simulink library "lib_transmission2"  (Simulink 10.1)
settings: Solver=VariableStepAuto  StartTime=0.0  StopTime=10.0  RelTol=1e-3
undefined symbols (not defined in the file or in its folder): cyc_mph, fc_map_spd, fc_max_trq, fc_spd_scale, fc_trq_scale, fd_inertia, fd_loss, fd_ratio, gb_gear_number_lookup, gb_gears_num, gb_inertia, gb_loss_const, gb_loss_input_spd_coeff, gb_loss_input_trq_coeff, gb_loss_output_spd_coeff, gb_loss_output_trq_coeff, gb_num_init, gb_ratio, gb_shift_delay, gb_spd_scale, gb_trq_scale, htc_inertia, htc_k_adv, htc_k_adv_coast, htc_lockup, htc_lockup_load, htc_lockup_spd, htc_lu_gear_range, htc_max_coast_tr, htc_min_coast_tr, htc_pump_loss_spd, htc_pump_loss_trq_lockup, htc_pump_loss_trq_unlock, htc_sr, htc_sr_coast, htc_tr, htc_tr_coast, htc_unlock_spd, mc_map_spd, mc_max_trq, mc_overtrq_factor, mc_spd_scale, mc_trq_scale, tc_loss, tc_mc_to_fc_ratio, tx_eff_map, tx_map_spd, tx_map_trq, tx_pg_r, tx_pg_s, tx_speed_dep, vc_clutch_bool, vc_idle_spd, vc_launch_spd, wh_radius
undefined symbols (not defined in the file): gb_dnshift_load, gb_dnshift_spd, gb_map_spd_out, gb_map_trq_in, gb_map_trq_out, gb_upshift_load, gb_upshift_spd, logFlag
libraries: lib_controls x1, lib_etc x1, lib_controls2 x1, lib_transmission x1
(part 14 of 17)

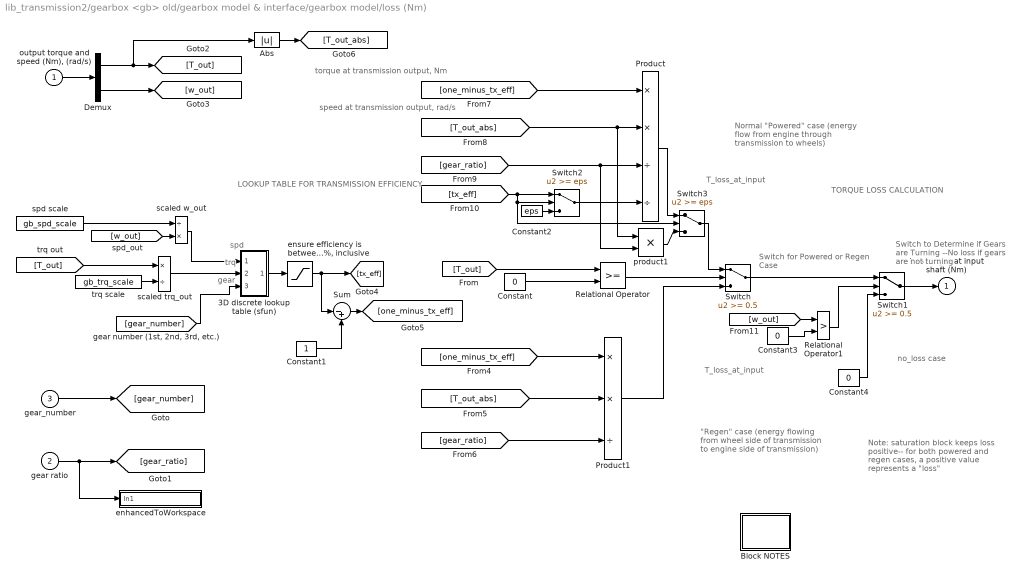
== system lib_transmission2/gearbox <gb> old/gearbox model & interface/gearbox model/loss (Nm) ==
  note: TORQUE LOSS CALCULATION
  note: gear
  note: trq
  note: spd
  note: torque at transmission output, Nm
  note: speed at transmission output, rad/s
  note: no_loss case
  note: Note: saturation block keeps
      | loss positive-- for both powered
      | and regen cases, a
      | positive value represents a "loss"
  note: Switch for Powered
      |  or Regen Case
  note: Switch to Determine
      | if Gears are Turning
      | --No loss if gears
      | are not turning
  note: Normal "Powered" case
      | (energy flow from engine
      | through transmission to wheels)
  note: T_loss_at_input
  note: "Regen" case
      | (energy flowing from
      | wheel side of transmission
      | to engine side of transmission)
  note: T_loss_at_input
  note: LOOKUP TABLE FOR TRANSMISSION EFFICIENCY
  "output torque and speed (Nm), (rad/s)" : Inport
  gear ratio : Inport  Port=2
  gear_number : Inport  Port=3
  3D discrete lookup table (sfun) : Subsystem  mask{tx_map_spd=tx_map_spd, tx_map_trq=tx_map_trq, tx_eff_map=tx_eff_map}
      mask prompts: tx_map_spd "Row Lookup"; tx_map_trq "Column Lookup"; tx_eff_map "Lookup Matrix"
  Abs : Abs  SaturateOnIntegerOverflow=on
  Block NOTES : Subsystem
      mask Display: disp('Block\nNOTES')
  Constant : Constant  Value=0
  Constant1 : Constant
  Constant2 : Constant  Value=eps
  Constant3 : Constant  Value=0
  Constant4 : Constant  Value=0
  Demux : Demux  Outputs=2
  Product : Product  Inputs=**//  SaturateOnIntegerOverflow=on
  Product1 : Product  Inputs=**/  SaturateOnIntegerOverflow=on
  Relational Operator : RelationalOperator  RndMeth=Nearest  InputSameDT=on
  Relational Operator1 : RelationalOperator  Operator=>  RndMeth=Nearest  InputSameDT=on
  Sum : Sum  Inputs=|-+  SaturateOnIntegerOverflow=on
  Switch : Switch  Threshold=0.5  SaturateOnIntegerOverflow=on  InputSameDT=on
  Switch1 : Switch  Threshold=0.5  SaturateOnIntegerOverflow=on  InputSameDT=on
  Switch2 : Switch  Threshold=eps  SaturateOnIntegerOverflow=on  InputSameDT=on
  Switch3 : Switch  Threshold=eps  SaturateOnIntegerOverflow=on  InputSameDT=on
  enhancedToWorkspace : Subsystem  TreatAsAtomicUnit=on  mask(enhancedToWorkspace){generalName=generalName, specificName=current_gear_ratio, logFlag=logFlag}
      mask prompts: generalName "General Name [char-evaluated]"; specificName "Specific Name [char-literal]"; logFlag "Enable flag (1=on,0=off)"
      mask help: A wrapper for the Simulink "To Workspace" block that allows you to evaluate the name of the variable to log to workspace. This is useful to avoid the double logging errors that occur when you pull in two library models that attempt to log to the same variable.
      mask init:
      | enhancedToWsMaker
      settings: CopyFcn=breakLinkCopyFcn  ParentCloseFcn=breakLinkParCloseFcn
      mask Help:
      | <h2>Enhanced To Workspace Block</h2>
      | <h3>Parameters</h3>
      | <UL>
      | <li><b>General Name:</b> This is the more general name of the variable. Variables are saved to the workspace as <i>generalName_specificName</i>. Note that this is an evaluated variable. If you would like to type in the value directly, it must be surrounded with single quotes. Otherwise you can input the name of a variable containing a char string.</li>
      | <li><b>Specific Name:</b> This is the specific name of the variable. Note that this is input as a char literal (i.e., you don't need quotes).</li>
      | <li><b>Enable Flag:</b> This flag should have the value of 0 or 1. If 0, the variable will not be logged to the workspace. If 1, the variable will be logged. This is done so that variable logging can be turned off to improve speed.</li>
      | </ul>
      | <h3>Overview</h3>
      | <p>The enhanced to workspace block was put together to allow one to dynamically resolve variable names at run time in simulink. This is most powerful when used in conjunction with a masked subsystem to allow multiple instances of that masked subsytem to be used in the same model. The strategy is to set the generalName in the block mask which will allow the block to change the general name for all variable logging on the fly.
      | <h3>Helper Files</h3>
      | <p>Three m-files are required by the enhancedToWorkspace block. These files are located in the &lt; ADVISOR root &gt;/GUI directory :
      | <ul>
      | <li><i>enhancedToWsMaker.m</i> This file runs the mask initialization for the block</li>
      | <li><i>breakLinkCopyFcn.m</i> This file is used by the block callback when the simulink block is copied. It is necessary to break the link to the enhancedToWorkspace similar to the To Workspace block in order for it to be able to configure itself. (Try copying simulink's To Workspace block--it is impossible to make a link)</li>
      | <li><i>breakLinkParCloseFcn.m</i> This file is similar to the breakLinkCopyFcn and is used when a parent system is closed</li>
      | </ul>
      | <hr>
      | 
      | <p>Created 2003-Jan-21, Michael Patrick O'Keefe, NREL</p>
      | 
      | <!--
      | <VARDEF>
      | <H3>var_name</H3>
      | <UL>
      | <LI><B>data type</B> data type here</LI>
      | <LI><B>units</B> units here</LI>
      | <LI><B>vehicle type</B> vehicle type here</LI>
      | <LI><B>description</B> description here</LI>
      | </UL>
      | </VARDEF>
      | -->
      mask Display: disp([generalName,'_',specificName])
  "ensure efficiency is between  0% and 100%, inclusive" : Saturate  UpperLimit=1  LowerLimit=0
  product1 : Product  SaturateOnIntegerOverflow=on
  scaled trq_out : Product  Inputs=*/  SaturateOnIntegerOverflow=on
  scaled w_out : Product  Inputs=/*  SaturateOnIntegerOverflow=on
  spd scale : Constant  Value=gb_spd_scale
  trq scale : Constant  Value=gb_trq_scale
  loss torque at input shaft (Nm) : Outport  InitialOutput=0
  wires:
  product1/1 -> Switch3/3
  Product/1 -> Switch3/1
  Switch3/1 -> Switch/1
  Constant2/1 -> Switch2/3
  [tx_eff] -> Switch3/2, Switch2/2, Switch2/1
  Switch2/1 -> Product/4
  gear_number/1 -> [gear_number]
  gear ratio/1 -> [gear_ratio], enhancedToWorkspace/1(In1)
  spd scale/1 -> scaled w_out/1
  [w_out] -> scaled w_out/2
  Sum/1 -> [one_minus_tx_eff]
  Constant1/1 -> Sum/2
  trq scale/1 -> scaled trq_out/2
  scaled trq_out/1 -> 3D discrete lookup table (sfun)/2(lookup trq (Nm))
  [T_out] -> scaled trq_out/1
  scaled w_out/1 -> 3D discrete lookup table (sfun)/1(lookup speed (rad/s))
  "ensure efficiency is between  0% and 100%, inclusive"/1 -> Sum/1, [tx_eff]
  3D discrete lookup table (sfun)/1(tx_eff) -> "ensure efficiency is between  0% and 100%, inclusive"/1
  Switch/1 -> Switch1/1
  Abs/1 -> [T_out_abs]
  Demux/1 -> Abs/1, [T_out]
  Relational Operator1/1 -> Switch1/2
  Constant3/1 -> Relational Operator1/2
  [w_out] -> Relational Operator1/1
  Constant4/1 -> Switch1/3
  Switch1/1 -> loss torque at input shaft (Nm)/1
  [gear_ratio] -> product1/2, Product/3
  [T_out_abs] -> product1/1, Product/2
  [one_minus_tx_eff] -> Product/1
  [T_out_abs] -> Product1/2
  [gear_ratio] -> Product1/3
  [one_minus_tx_eff] -> Product1/1
  Product1/1 -> Switch/3
  [T_out] -> Relational Operator/1
  Constant/1 -> Relational Operator/2
  Relational Operator/1 -> Switch/2
  [gear_number] -> 3D discrete lookup table (sfun)/3("gear_number  (e.g., 1, 2, 3)")
  Demux/2 -> [w_out]
  "output torque and speed (Nm), (rad/s)"/1 -> Demux/1

== system lib_transmission2/hydraulic torque converter <htc>/conventional HTC  and Interface/htc model/SR ==
  T,w req out : Inport
  w in : Inport  Port=2
  >0 : Saturate  UpperLimit=inf  LowerLimit=eps
  Constant : Constant  Value=0
  Constant1 : Constant  Value=vc_idle_spd+eps
  Constant3 : Constant
  K_adv : Subsystem
  K_adv_coast : Subsystem
  Logical Operator : Logic  Operator=NOT  Inputs=1
  Logical Operator1 : Logic  Operator=NOT  Inputs=1
  MinMax : MinMax  Inputs=2
  Relational Operator : RelationalOperator  RndMeth=Nearest  InputSameDT=on
  SR Look-Up Table SR=wout/win : Lookup  InputValues=htc_k_adv  Table=htc_sr  SaturateOnIntegerOverflow=on
  SR Look-Up Table SR=wout/win coast : Lookup  InputValues=fliplr(htc_k_adv_coast)  Table=fliplr(htc_sr_coast)  SaturateOnIntegerOverflow=on
  SRmax= wout/win,min : Product  Inputs=*/  SaturateOnIntegerOverflow=on
  T : Selector  InputPortWidth=2  IndexOptions=Index vector (dialog)  Indices=1  OutputSizes=1
  enhancedToWorkspace1 : Subsystem  TreatAsAtomicUnit=on  mask(enhancedToWorkspace){generalName=generalName, specificName=coasting, logFlag=logFlag}
      mask prompts: generalName "General Name [char-evaluated]"; specificName "Specific Name [char-literal]"; logFlag "Enable flag (1=on,0=off)"
      mask help: A wrapper for the Simulink "To Workspace" block that allows you to evaluate the name of the variable to log to workspace. This is useful to avoid the double logging errors that occur when you pull in two library models that attempt to log to the same variable.
      mask init:
      | enhancedToWsMaker
      settings: CopyFcn=breakLinkCopyFcn  ParentCloseFcn=breakLinkParCloseFcn
      mask Help:
      | <h2>Enhanced To Workspace Block</h2>
      | <h3>Parameters</h3>
      | <UL>
      | <li><b>General Name:</b> This is the more general name of the variable. Variables are saved to the workspace as <i>generalName_specificName</i>. Note that this is an evaluated variable. If you would like to type in the value directly, it must be surrounded with single quotes. Otherwise you can input the name of a variable containing a char string.</li>
      | <li><b>Specific Name:</b> This is the specific name of the variable. Note that this is input as a char literal (i.e., you don't need quotes).</li>
      | <li><b>Enable Flag:</b> This flag should have the value of 0 or 1. If 0, the variable will not be logged to the workspace. If 1, the variable will be logged. This is done so that variable logging can be turned off to improve speed.</li>
      | </ul>
      | <h3>Overview</h3>
      | <p>The enhanced to workspace block was put together to allow one to dynamically resolve variable names at run time in simulink. This is most powerful when used in conjunction with a masked subsystem to allow multiple instances of that masked subsytem to be used in the same model. The strategy is to set the generalName in the block mask which will allow the block to change the general name for all variable logging on the fly.
      | <h3>Helper Files</h3>
      | <p>Three m-files are required by the enhancedToWorkspace block. These files are located in the &lt; ADVISOR root &gt;/GUI directory :
      | <ul>
      | <li><i>enhancedToWsMaker.m</i> This file runs the mask initialization for the block</li>
      | <li><i>breakLinkCopyFcn.m</i> This file is used by the block callback when the simulink block is copied. It is necessary to break the link to the enhancedToWorkspace similar to the To Workspace block in order for it to be able to configure itself. (Try copying simulink's To Workspace block--it is impossible to make a link)</li>
      | <li><i>breakLinkParCloseFcn.m</i> This file is similar to the breakLinkCopyFcn and is used when a parent system is closed</li>
      | </ul>
      | <hr>
      | 
      | <p>Created 2003-Jan-21, Michael Patrick O'Keefe, NREL</p>
      | 
      | <!--
      | <VARDEF>
      | <H3>var_name</H3>
      | <UL>
      | <LI><B>data type</B> data type here</LI>
      | <LI><B>units</B> units here</LI>
      | <LI><B>vehicle type</B> vehicle type here</LI>
      | <LI><B>description</B> description here</LI>
      | </UL>
      | </VARDEF>
      | -->
      mask Display: disp([generalName,'_',specificName])
  enhancedToWorkspace2 : Subsystem  TreatAsAtomicUnit=on  mask(enhancedToWorkspace){generalName=generalName, specificName=locked, logFlag=logFlag}
      mask prompts: generalName "General Name [char-evaluated]"; specificName "Specific Name [char-literal]"; logFlag "Enable flag (1=on,0=off)"
      mask help: A wrapper for the Simulink "To Workspace" block that allows you to evaluate the name of the variable to log to workspace. This is useful to avoid the double logging errors that occur when you pull in two library models that attempt to log to the same variable.
      mask init:
      | enhancedToWsMaker
      settings: CopyFcn=breakLinkCopyFcn  ParentCloseFcn=breakLinkParCloseFcn
      mask Help:
      | <h2>Enhanced To Workspace Block</h2>
      | <h3>Parameters</h3>
      | <UL>
      | <li><b>General Name:</b> This is the more general name of the variable. Variables are saved to the workspace as <i>generalName_specificName</i>. Note that this is an evaluated variable. If you would like to type in the value directly, it must be surrounded with single quotes. Otherwise you can input the name of a variable containing a char string.</li>
      | <li><b>Specific Name:</b> This is the specific name of the variable. Note that this is input as a char literal (i.e., you don't need quotes).</li>
      | <li><b>Enable Flag:</b> This flag should have the value of 0 or 1. If 0, the variable will not be logged to the workspace. If 1, the variable will be logged. This is done so that variable logging can be turned off to improve speed.</li>
      | </ul>
      | <h3>Overview</h3>
      | <p>The enhanced to workspace block was put together to allow one to dynamically resolve variable names at run time in simulink. This is most powerful when used in conjunction with a masked subsystem to allow multiple instances of that masked subsytem to be used in the same model. The strategy is to set the generalName in the block mask which will allow the block to change the general name for all variable logging on the fly.
      | <h3>Helper Files</h3>
      | <p>Three m-files are required by the enhancedToWorkspace block. These files are located in the &lt; ADVISOR root &gt;/GUI directory :
      | <ul>
      | <li><i>enhancedToWsMaker.m</i> This file runs the mask initialization for the block</li>
      | <li><i>breakLinkCopyFcn.m</i> This file is used by the block callback when the simulink block is copied. It is necessary to break the link to the enhancedToWorkspace similar to the To Workspace block in order for it to be able to configure itself. (Try copying simulink's To Workspace block--it is impossible to make a link)</li>
      | <li><i>breakLinkParCloseFcn.m</i> This file is similar to the breakLinkCopyFcn and is used when a parent system is closed</li>
      | </ul>
      | <hr>
      | 
      | <p>Created 2003-Jan-21, Michael Patrick O'Keefe, NREL</p>
      | 
      | <!--
      | <VARDEF>
      | <H3>var_name</H3>
      | <UL>
      | <LI><B>data type</B> data type here</LI>
      | <LI><B>units</B> units here</LI>
      | <LI><B>vehicle type</B> vehicle type here</LI>
      | <LI><B>description</B> description here</LI>
      | </UL>
      | </VARDEF>
      | -->
      mask Display: disp([generalName,'_',specificName])
  if coasting : Switch  Threshold=eps  SaturateOnIntegerOverflow=on  InputSameDT=on
  "locked up, then SR=1" : Switch  Threshold=eps  SaturateOnIntegerOverflow=on  InputSameDT=on
  min,max : Saturate  UpperLimit=inf  LowerLimit=1
  shifting SR : Subsystem
  wout,req : Selector  InputPortWidth=2  IndexOptions=Index vector (dialog)  Indices=2  OutputSizes=1
  SR : Outport  InitialOutput=0
  coasting : Outport  Port=2  InitialOutput=0
  wires:
  K_adv/1(K_adv) -> SR Look-Up Table SR=wout/win/1
  Logical Operator1/1 -> coasting/1, enhancedToWorkspace1/1(In1)
  >0/1 -> SR/1
  if coasting/1 -> >0/1
  K_adv_coast/1(K_adv_coast) -> SR Look-Up Table SR=wout/win coast/1
  MinMax/1 -> if coasting/3
  min,max/1 -> MinMax/1
  wout,req/1 -> SRmax= wout/win,min/1
  Constant1/1 -> SRmax= wout/win,min/2
  SRmax= wout/win,min/1 -> MinMax/2
  shifting SR/1(SR limited) -> if coasting/1
  "locked up, then SR=1"/1 -> shifting SR/3(SR)
  w in/1 -> shifting SR/2(w in)
  SR Look-Up Table SR=wout/win/1 -> "locked up, then SR=1"/1
  Constant3/1 -> "locked up, then SR=1"/3
  Logical Operator/1 -> "locked up, then SR=1"/2
  Relational Operator/1 -> Logical Operator1/1, if coasting/2
  T/1 -> Relational Operator/1
  Constant/1 -> Relational Operator/2
  SR Look-Up Table SR=wout/win coast/1 -> min,max/1
  T,w req out/1 -> shifting SR/1(T,w req out), K_adv/1("Req'd output trq and spd (Nm), (rad/s)"), wout,req/1, K_adv_coast/1("Req'd output trq and spd (Nm), (rad/s)"), T/1
  [locked_up] -> Logical Operator/1, enhancedToWorkspace2/1(In1)

== system lib_transmission2/hydraulic torque converter <htc>/conventional HTC  and Interface/htc model/T, shifting ==
  TR : Inport
  Req'd  input trq : Inport  Port=2
  Req'd output trq : Inport  Port=3
  htc_spd_in_a : Inport  Port=4
  SR : Inport  Port=5
  Memory : Memory
  Memory1 : Memory
  MinMax : MinMax  Inputs=2
  TR Look-Up Table TR=Tout/Tin : Lookup  InputValues=htc_sr  Table=htc_tr  SaturateOnIntegerOverflow=on
  T_max : Subsystem
  Tin*TR= Tout,req : Product  SaturateOnIntegerOverflow=on
  engine speed estimator : Subsystem
  "shifting, override zero Trequest" : Switch  Threshold=eps  SaturateOnIntegerOverflow=on  InputSameDT=on
  T req : Outport
  wires:
  Tin*TR= Tout,req/1 -> Memory/1
  TR/1 -> Tin*TR= Tout,req/2
  Req'd  input trq/1 -> Tin*TR= Tout,req/1
  Memory/1 -> "shifting, override zero Trequest"/1
  T_max/1(T_max max gain from htc) -> MinMax/2
  "shifting, override zero Trequest"/1 -> MinMax/1
  TR Look-Up Table TR=Tout/Tin/1 -> T_max/2(TR)
  MinMax/1 -> T req/1
  engine speed estimator/1(Out1) -> T_max/1(w_APU)
  Memory1/1 -> TR Look-Up Table TR=Tout/Tin/1
  SR/1 -> Memory1/1
  htc_spd_in_a/1 -> engine speed estimator/1(htc_spd_in_a)
  Req'd output trq/1 -> "shifting, override zero Trequest"/3
  [shifting] -> "shifting, override zero Trequest"/2

== system lib_transmission2/hydraulic torque converter <htc>/conventional HTC  and Interface/htc model/TR ==
  SR : Inport
  coasting : Inport  Port=2
  1/SR*TR  for coast : Fcn  Expr=1/u
  Constant3 : Constant
  Logical Operator : Logic  Operator=NOT  Inputs=1
  Logical Operator1 : Logic  Operator=NOT  Inputs=1
  TR Look-Up Table TR=Tout/Tin : Lookup  InputValues=htc_sr  Table=htc_tr  SaturateOnIntegerOverflow=on
  TR Look-Up Table TR=Tout/Tin coast : Lookup  InputValues=htc_sr_coast  Table=htc_tr_coast  SaturateOnIntegerOverflow=on
  effic=SR*TR : Product  Inputs=**  SaturateOnIntegerOverflow=on
  enhancedToWorkspace2 : Subsystem  TreatAsAtomicUnit=on  mask(enhancedToWorkspace){generalName=generalName, specificName=efficiency, logFlag=logFlag}
      mask prompts: generalName "General Name [char-evaluated]"; specificName "Specific Name [char-literal]"; logFlag "Enable flag (1=on,0=off)"
      mask help: A wrapper for the Simulink "To Workspace" block that allows you to evaluate the name of the variable to log to workspace. This is useful to avoid the double logging errors that occur when you pull in two library models that attempt to log to the same variable.
      mask init:
      | enhancedToWsMaker
      settings: CopyFcn=breakLinkCopyFcn  ParentCloseFcn=breakLinkParCloseFcn
      mask Help:
      | <h2>Enhanced To Workspace Block</h2>
      | <h3>Parameters</h3>
      | <UL>
      | <li><b>General Name:</b> This is the more general name of the variable. Variables are saved to the workspace as <i>generalName_specificName</i>. Note that this is an evaluated variable. If you would like to type in the value directly, it must be surrounded with single quotes. Otherwise you can input the name of a variable containing a char string.</li>
      | <li><b>Specific Name:</b> This is the specific name of the variable. Note that this is input as a char literal (i.e., you don't need quotes).</li>
      | <li><b>Enable Flag:</b> This flag should have the value of 0 or 1. If 0, the variable will not be logged to the workspace. If 1, the variable will be logged. This is done so that variable logging can be turned off to improve speed.</li>
      | </ul>
      | <h3>Overview</h3>
      | <p>The enhanced to workspace block was put together to allow one to dynamically resolve variable names at run time in simulink. This is most powerful when used in conjunction with a masked subsystem to allow multiple instances of that masked subsytem to be used in the same model. The strategy is to set the generalName in the block mask which will allow the block to change the general name for all variable logging on the fly.
      | <h3>Helper Files</h3>
      | <p>Three m-files are required by the enhancedToWorkspace block. These files are located in the &lt; ADVISOR root &gt;/GUI directory :
      | <ul>
      | <li><i>enhancedToWsMaker.m</i> This file runs the mask initialization for the block</li>
      | <li><i>breakLinkCopyFcn.m</i> This file is used by the block callback when the simulink block is copied. It is necessary to break the link to the enhancedToWorkspace similar to the To Workspace block in order for it to be able to configure itself. (Try copying simulink's To Workspace block--it is impossible to make a link)</li>
      | <li><i>breakLinkParCloseFcn.m</i> This file is similar to the breakLinkCopyFcn and is used when a parent system is closed</li>
      | </ul>
      | <hr>
      | 
      | <p>Created 2003-Jan-21, Michael Patrick O'Keefe, NREL</p>
      | 
      | <!--
      | <VARDEF>
      | <H3>var_name</H3>
      | <UL>
      | <LI><B>data type</B> data type here</LI>
      | <LI><B>units</B> units here</LI>
      | <LI><B>vehicle type</B> vehicle type here</LI>
      | <LI><B>description</B> description here</LI>
      | </UL>
      | </VARDEF>
      | -->
      mask Display: disp([generalName,'_',specificName])
  if coasting : Switch  Threshold=eps  SaturateOnIntegerOverflow=on  InputSameDT=on
  if coasting1 : Switch  Threshold=eps  SaturateOnIntegerOverflow=on  InputSameDT=on
  "locked up, then TR=1" : Switch  Threshold=eps  SaturateOnIntegerOverflow=on  InputSameDT=on
  min,max : Saturate  UpperLimit=htc_max_coast_tr  LowerLimit=htc_min_coast_tr
  TR : Outport  InitialOutput=0
  tag scope: htc_efficiency=scoped
  wires:
  if coasting1/1 -> [htc_efficiency], enhancedToWorkspace2/1(In1)
  1/SR*TR  for coast/1 -> if coasting1/3
  effic=SR*TR/1 -> 1/SR*TR  for coast/1, if coasting1/1
  Logical Operator1/1 -> if coasting1/2, if coasting/2
  if coasting/1 -> effic=SR*TR/2, TR/1
  coasting/1 -> Logical Operator1/1
  SR/1 -> effic=SR*TR/1, TR Look-Up Table TR=Tout/Tin/1, TR Look-Up Table TR=Tout/Tin coast/1
  min,max/1 -> if coasting/3
  TR Look-Up Table TR=Tout/Tin coast/1 -> min,max/1
  "locked up, then TR=1"/1 -> if coasting/1
  Logical Operator/1 -> "locked up, then TR=1"/2
  [locked_up] -> Logical Operator/1
  Constant3/1 -> "locked up, then TR=1"/3
  TR Look-Up Table TR=Tout/Tin/1 -> "locked up, then TR=1"/1

== system lib_transmission2/hydraulic torque converter <htc>/conventional HTC  and Interface/htc model/effect of inertia (Nm) ==
  note: This block computes the torque required to overcome the inertia of the
      | turbine (plus 1/2 fluid in htc).
  turbine/output speed (rad/s) : Inport
  Constant : Constant  Value=htc_inertia
  Product : Product  SaturateOnIntegerOverflow=on
  d/dt : Derivative
  inertia torque (Nm) : Outport  InitialOutput=0
  wires:
  Product/1 -> inertia torque (Nm)/1
  Constant/1 -> Product/2
  turbine/output speed (rad/s)/1 -> d/dt/1
  d/dt/1 -> Product/1

== system lib_transmission2/hydraulic torque converter <htc>/conventional HTC  and Interface/htc model/enhancedToWorkspace ==
  In1 : Inport
  To Workspace : ToWorkspace  VariableName=htc_trq_in_a  SampleTime=-1
  wires:
  In1/1 -> To Workspace/1

== system lib_transmission2/hydraulic torque converter <htc>/conventional HTC  and Interface/htc model/enhancedToWorkspace1 ==
  In1 : Inport
  To Workspace : ToWorkspace  VariableName=htc_spd_in_a  SampleTime=-1
  wires:
  In1/1 -> To Workspace/1

== system lib_transmission2/hydraulic torque converter <htc>/conventional HTC  and Interface/htc model/enhancedToWorkspace10 ==
  In1 : Inport
  To Workspace : ToWorkspace  VariableName=htc_spd_out_a  SampleTime=-1
  wires:
  In1/1 -> To Workspace/1

== system lib_transmission2/hydraulic torque converter <htc>/conventional HTC  and Interface/htc model/enhancedToWorkspace2 ==
  In1 : Inport
  To Workspace : ToWorkspace  VariableName=htc_trq_out_r  SampleTime=-1
  wires:
  In1/1 -> To Workspace/1

== system lib_transmission2/hydraulic torque converter <htc>/conventional HTC  and Interface/htc model/enhancedToWorkspace3 ==
  In1 : Inport
  To Workspace : ToWorkspace  VariableName=htc_spd_out_r  SampleTime=-1
  wires:
  In1/1 -> To Workspace/1

== system lib_transmission2/hydraulic torque converter <htc>/conventional HTC  and Interface/htc model/enhancedToWorkspace4 ==
  In1 : Inport
  To Workspace : ToWorkspace  VariableName=htc_sr_hist  SampleTime=-1
  wires:
  In1/1 -> To Workspace/1

== system lib_transmission2/hydraulic torque converter <htc>/conventional HTC  and Interface/htc model/enhancedToWorkspace5 ==
  In1 : Inport
  To Workspace : ToWorkspace  VariableName=htc_tr_hist  SampleTime=-1
  wires:
  In1/1 -> To Workspace/1

== system lib_transmission2/hydraulic torque converter <htc>/conventional HTC  and Interface/htc model/enhancedToWorkspace6 ==
  In1 : Inport
  To Workspace : ToWorkspace  VariableName=htc_spd_in_r  SampleTime=-1
  wires:
  In1/1 -> To Workspace/1

== system lib_transmission2/hydraulic torque converter <htc>/conventional HTC  and Interface/htc model/enhancedToWorkspace7 ==
  In1 : Inport
  To Workspace : ToWorkspace  VariableName=htc_trq_in_r  SampleTime=-1
  wires:
  In1/1 -> To Workspace/1

== system lib_transmission2/hydraulic torque converter <htc>/conventional HTC  and Interface/htc model/enhancedToWorkspace8 ==
  In1 : Inport
  To Workspace : ToWorkspace  VariableName=htc_trq_inertia  SampleTime=-1
  wires:
  In1/1 -> To Workspace/1

== system lib_transmission2/hydraulic torque converter <htc>/conventional HTC  and Interface/htc model/enhancedToWorkspace9 ==
  In1 : Inport
  To Workspace : ToWorkspace  VariableName=htc_trq_out_a  SampleTime=-1
  wires:
  In1/1 -> To Workspace/1

== system lib_transmission2/hydraulic torque converter <htc> HEV/HTC for parallel HEV and Interface/model for parallel HEV/Block NOTES ==
  note: This block predicts the relative speed of the HTC input (pump) and output
      | (turbine).  Torque converter lockup is modeled.

== system lib_transmission2/hydraulic torque converter <htc> HEV/HTC for parallel HEV and Interface/model for parallel HEV/SR ==
  T,w req out : Inport
  w in : Inport  Port=2
  >0 : Saturate  UpperLimit=inf  LowerLimit=eps
  Constant : Constant  Value=0
  Constant1 : Constant  Value=vc_idle_spd+eps
  Constant3 : Constant
  K_adv : Subsystem
  K_adv_coast : Subsystem
  Logical Operator : Logic  Operator=NOT  Inputs=1
  Logical Operator1 : Logic  Operator=NOT  Inputs=1
  MinMax : MinMax  Inputs=2
  Relational Operator : RelationalOperator  RndMeth=Nearest  InputSameDT=on
  SR Look-Up Table SR=wout/win : Lookup  InputValues=htc_k_adv  Table=htc_sr  SaturateOnIntegerOverflow=on
  SR Look-Up Table SR=wout/win coast : Lookup  InputValues=fliplr(htc_k_adv_coast)  Table=fliplr(htc_sr_coast)  SaturateOnIntegerOverflow=on
  SRmax= wout/win,min : Product  Inputs=*/  SaturateOnIntegerOverflow=on
  T : Selector  InputPortWidth=2  IndexOptions=Index vector (dialog)  Indices=1  OutputSizes=1
  enhancedToWorkspace : Subsystem  TreatAsAtomicUnit=on  mask(enhancedToWorkspace){generalName=generalName, specificName=locked, logFlag=logFlag}
      mask prompts: generalName "General Name [char-evaluated]"; specificName "Specific Name [char-literal]"; logFlag "Enable flag (1=on,0=off)"
      mask help: A wrapper for the Simulink "To Workspace" block that allows you to evaluate the name of the variable to log to workspace. This is useful to avoid the double logging errors that occur when you pull in two library models that attempt to log to the same variable.
      mask init:
      | enhancedToWsMaker
      settings: CopyFcn=breakLinkCopyFcn  ParentCloseFcn=breakLinkParCloseFcn
      mask Help:
      | <h2>Enhanced To Workspace Block</h2>
      | <h3>Parameters</h3>
      | <UL>
      | <li><b>General Name:</b> This is the more general name of the variable. Variables are saved to the workspace as <i>generalName_specificName</i>. Note that this is an evaluated variable. If you would like to type in the value directly, it must be surrounded with single quotes. Otherwise you can input the name of a variable containing a char string.</li>
      | <li><b>Specific Name:</b> This is the specific name of the variable. Note that this is input as a char literal (i.e., you don't need quotes).</li>
      | <li><b>Enable Flag:</b> This flag should have the value of 0 or 1. If 0, the variable will not be logged to the workspace. If 1, the variable will be logged. This is done so that variable logging can be turned off to improve speed.</li>
      | </ul>
      | <h3>Overview</h3>
      | <p>The enhanced to workspace block was put together to allow one to dynamically resolve variable names at run time in simulink. This is most powerful when used in conjunction with a masked subsystem to allow multiple instances of that masked subsytem to be used in the same model. The strategy is to set the generalName in the block mask which will allow the block to change the general name for all variable logging on the fly.
      | <h3>Helper Files</h3>
      | <p>Three m-files are required by the enhancedToWorkspace block. These files are located in the &lt; ADVISOR root &gt;/GUI directory :
      | <ul>
      | <li><i>enhancedToWsMaker.m</i> This file runs the mask initialization for the block</li>
      | <li><i>breakLinkCopyFcn.m</i> This file is used by the block callback when the simulink block is copied. It is necessary to break the link to the enhancedToWorkspace similar to the To Workspace block in order for it to be able to configure itself. (Try copying simulink's To Workspace block--it is impossible to make a link)</li>
      | <li><i>breakLinkParCloseFcn.m</i> This file is similar to the breakLinkCopyFcn and is used when a parent system is closed</li>
      | </ul>
      | <hr>
      | 
      | <p>Created 2003-Jan-21, Michael Patrick O'Keefe, NREL</p>
      | 
      | <!--
      | <VARDEF>
      | <H3>var_name</H3>
      | <UL>
      | <LI><B>data type</B> data type here</LI>
      | <LI><B>units</B> units here</LI>
      | <LI><B>vehicle type</B> vehicle type here</LI>
      | <LI><B>description</B> description here</LI>
      | </UL>
      | </VARDEF>
      | -->
      mask Display: disp([generalName,'_',specificName])
  enhancedToWorkspace1 : Subsystem  TreatAsAtomicUnit=on  mask(enhancedToWorkspace){generalName=generalName, specificName=coasting, logFlag=logFlag}
      mask prompts: generalName "General Name [char-evaluated]"; specificName "Specific Name [char-literal]"; logFlag "Enable flag (1=on,0=off)"
      mask help: A wrapper for the Simulink "To Workspace" block that allows you to evaluate the name of the variable to log to workspace. This is useful to avoid the double logging errors that occur when you pull in two library models that attempt to log to the same variable.
      mask init:
      | enhancedToWsMaker
      settings: CopyFcn=breakLinkCopyFcn  ParentCloseFcn=breakLinkParCloseFcn
      mask Help:
      | <h2>Enhanced To Workspace Block</h2>
      | <h3>Parameters</h3>
      | <UL>
      | <li><b>General Name:</b> This is the more general name of the variable. Variables are saved to the workspace as <i>generalName_specificName</i>. Note that this is an evaluated variable. If you would like to type in the value directly, it must be surrounded with single quotes. Otherwise you can input the name of a variable containing a char string.</li>
      | <li><b>Specific Name:</b> This is the specific name of the variable. Note that this is input as a char literal (i.e., you don't need quotes).</li>
      | <li><b>Enable Flag:</b> This flag should have the value of 0 or 1. If 0, the variable will not be logged to the workspace. If 1, the variable will be logged. This is done so that variable logging can be turned off to improve speed.</li>
      | </ul>
      | <h3>Overview</h3>
      | <p>The enhanced to workspace block was put together to allow one to dynamically resolve variable names at run time in simulink. This is most powerful when used in conjunction with a masked subsystem to allow multiple instances of that masked subsytem to be used in the same model. The strategy is to set the generalName in the block mask which will allow the block to change the general name for all variable logging on the fly.
      | <h3>Helper Files</h3>
      | <p>Three m-files are required by the enhancedToWorkspace block. These files are located in the &lt; ADVISOR root &gt;/GUI directory :
      | <ul>
      | <li><i>enhancedToWsMaker.m</i> This file runs the mask initialization for the block</li>
      | <li><i>breakLinkCopyFcn.m</i> This file is used by the block callback when the simulink block is copied. It is necessary to break the link to the enhancedToWorkspace similar to the To Workspace block in order for it to be able to configure itself. (Try copying simulink's To Workspace block--it is impossible to make a link)</li>
      | <li><i>breakLinkParCloseFcn.m</i> This file is similar to the breakLinkCopyFcn and is used when a parent system is closed</li>
      | </ul>
      | <hr>
      | 
      | <p>Created 2003-Jan-21, Michael Patrick O'Keefe, NREL</p>
      | 
      | <!--
      | <VARDEF>
      | <H3>var_name</H3>
      | <UL>
      | <LI><B>data type</B> data type here</LI>
      | <LI><B>units</B> units here</LI>
      | <LI><B>vehicle type</B> vehicle type here</LI>
      | <LI><B>description</B> description here</LI>
      | </UL>
      | </VARDEF>
      | -->
      mask Display: disp([generalName,'_',specificName])
  if coasting : Switch  Threshold=eps  SaturateOnIntegerOverflow=on  InputSameDT=on
  "locked up, then SR=1" : Switch  Threshold=eps  SaturateOnIntegerOverflow=on  InputSameDT=on
  min,max : Saturate  UpperLimit=inf  LowerLimit=1
  shifting SR : Subsystem
  wout,req : Selector  InputPortWidth=2  IndexOptions=Index vector (dialog)  Indices=2  OutputSizes=1
  SR : Outport  InitialOutput=0
  coasting : Outport  Port=2  InitialOutput=0
  wires:
  K_adv/1(K_adv) -> SR Look-Up Table SR=wout/win/1
  Logical Operator1/1 -> coasting/1, enhancedToWorkspace1/1(In1)
  >0/1 -> SR/1
  if coasting/1 -> >0/1
  K_adv_coast/1(K_adv_coast) -> SR Look-Up Table SR=wout/win coast/1
  MinMax/1 -> if coasting/3
  min,max/1 -> MinMax/1
  wout,req/1 -> SRmax= wout/win,min/1
  Constant1/1 -> SRmax= wout/win,min/2
  SRmax= wout/win,min/1 -> MinMax/2
  shifting SR/1(SR limited) -> if coasting/1
  "locked up, then SR=1"/1 -> shifting SR/3(SR)
  w in/1 -> shifting SR/2(w in)
  SR Look-Up Table SR=wout/win/1 -> "locked up, then SR=1"/1
  Constant3/1 -> "locked up, then SR=1"/3
  Logical Operator/1 -> "locked up, then SR=1"/2
  T/1 -> Relational Operator/1
  Constant/1 -> Relational Operator/2
  SR Look-Up Table SR=wout/win coast/1 -> min,max/1
  T,w req out/1 -> shifting SR/1(T,w req out), K_adv/1("Req'd output trq and spd (Nm), (rad/s)"), wout,req/1, K_adv_coast/1("Req'd output trq and spd (Nm), (rad/s)"), T/1
  [locked_up] -> Logical Operator/1, enhancedToWorkspace/1(In1)
  Relational Operator/1 -> Logical Operator1/1, if coasting/2

== system lib_transmission2/hydraulic torque converter <htc> HEV/HTC for parallel HEV and Interface/model for parallel HEV/T, shifting ==
  TR : Inport
  Req'd  input trq : Inport  Port=2
  Req'd output trq : Inport  Port=3
  htc_spd_in_a : Inport  Port=4
  SR : Inport  Port=5
  Memory : Memory
  Memory1 : Memory
  MinMax : MinMax  Inputs=2
  TR Look-Up Table TR=Tout/Tin : Lookup  InputValues=htc_sr  Table=htc_tr  SaturateOnIntegerOverflow=on
  T_max : Subsystem
  Tin*TR= Tout,req : Product  SaturateOnIntegerOverflow=on
  engine speed estimator : Subsystem
  "shifting, override zero Trequest" : Switch  Threshold=eps  SaturateOnIntegerOverflow=on  InputSameDT=on
  T req : Outport
  wires:
  Tin*TR= Tout,req/1 -> Memory/1
  TR/1 -> Tin*TR= Tout,req/2
  Req'd  input trq/1 -> Tin*TR= Tout,req/1
  Memory/1 -> "shifting, override zero Trequest"/1
  T_max/1(T_max max gain from htc) -> MinMax/2
  "shifting, override zero Trequest"/1 -> MinMax/1
  TR Look-Up Table TR=Tout/Tin/1 -> T_max/2(TR)
  MinMax/1 -> T req/1
  engine speed estimator/1(Out1) -> T_max/1(w_APU)
  Memory1/1 -> TR Look-Up Table TR=Tout/Tin/1
  SR/1 -> Memory1/1
  htc_spd_in_a/1 -> engine speed estimator/1(htc_spd_in_a)
  Req'd output trq/1 -> "shifting, override zero Trequest"/3
  [shifting] -> "shifting, override zero Trequest"/2

== system lib_transmission2/hydraulic torque converter <htc> HEV/HTC for parallel HEV and Interface/model for parallel HEV/TR ==
  SR : Inport
  coasting : Inport  Port=2
  1/SR*TR  for coast : Fcn  Expr=1/u
  Constant3 : Constant
  Logical Operator : Logic  Operator=NOT  Inputs=1
  Logical Operator1 : Logic  Operator=NOT  Inputs=1
  TR Look-Up Table TR=Tout/Tin : Lookup  InputValues=htc_sr  Table=htc_tr  SaturateOnIntegerOverflow=on
  TR Look-Up Table TR=Tout/Tin coast : Lookup  InputValues=htc_sr_coast  Table=htc_tr_coast  SaturateOnIntegerOverflow=on
  To Workspace11 : ToWorkspace  VariableName=htc_efficiency  SampleTime=-1
  effic=SR*TR : Product  Inputs=**  SaturateOnIntegerOverflow=on
  if coasting : Switch  Threshold=eps  SaturateOnIntegerOverflow=on  InputSameDT=on
  if coasting1 : Switch  Threshold=eps  SaturateOnIntegerOverflow=on  InputSameDT=on
  "locked up, then TR=1" : Switch  Threshold=eps  SaturateOnIntegerOverflow=on  InputSameDT=on
  min,max : Saturate  UpperLimit=htc_max_coast_tr  LowerLimit=htc_min_coast_tr
  TR : Outport  InitialOutput=0
  wires:
  if coasting1/1 -> To Workspace11/1
  1/SR*TR  for coast/1 -> if coasting1/3
  effic=SR*TR/1 -> 1/SR*TR  for coast/1, if coasting1/1
  Logical Operator1/1 -> if coasting1/2, if coasting/2
  if coasting/1 -> effic=SR*TR/2, TR/1
  coasting/1 -> Logical Operator1/1
  SR/1 -> effic=SR*TR/1, TR Look-Up Table TR=Tout/Tin/1, TR Look-Up Table TR=Tout/Tin coast/1
  min,max/1 -> if coasting/3
  TR Look-Up Table TR=Tout/Tin coast/1 -> min,max/1
  "locked up, then TR=1"/1 -> if coasting/1
  Logical Operator/1 -> "locked up, then TR=1"/2
  [locked_up] -> Logical Operator/1
  Constant3/1 -> "locked up, then TR=1"/3
  TR Look-Up Table TR=Tout/Tin/1 -> "locked up, then TR=1"/1

== system lib_transmission2/hydraulic torque converter <htc> HEV/HTC for parallel HEV and Interface/model for parallel HEV/effect of inertia (Nm) ==
  note: This block computes the torque required to overcome the inertia of the
      | turbine (plus 1/2 fluid in htc).
  turbine/output speed (rad/s) : Inport
  Constant : Constant  Value=htc_inertia
  Product : Product  SaturateOnIntegerOverflow=on
  d/dt : Derivative
  inertia torque (Nm) : Outport  InitialOutput=0
  wires:
  Product/1 -> inertia torque (Nm)/1
  Constant/1 -> Product/2
  turbine/output speed (rad/s)/1 -> d/dt/1
  d/dt/1 -> Product/1

== system lib_transmission2/hydraulic torque converter <htc> HEV/HTC for parallel HEV and Interface/model for parallel HEV/enhancedToWorkspace ==
  In1 : Inport
  Terminator : Terminator
  wires:
  In1/1 -> Terminator/1

== system lib_transmission2/hydraulic torque converter <htc> HEV/HTC for parallel HEV and Interface/model for parallel HEV/enhancedToWorkspace1 ==
  In1 : Inport
  Terminator : Terminator
  wires:
  In1/1 -> Terminator/1

== system lib_transmission2/hydraulic torque converter <htc> HEV/HTC for parallel HEV and Interface/model for parallel HEV/enhancedToWorkspace10 ==
  In1 : Inport
  Terminator : Terminator
  wires:
  In1/1 -> Terminator/1

== system lib_transmission2/hydraulic torque converter <htc> HEV/HTC for parallel HEV and Interface/model for parallel HEV/enhancedToWorkspace2 ==
  In1 : Inport
  Terminator : Terminator
  wires:
  In1/1 -> Terminator/1

== system lib_transmission2/hydraulic torque converter <htc> HEV/HTC for parallel HEV and Interface/model for parallel HEV/enhancedToWorkspace3 ==
  In1 : Inport
  Terminator : Terminator
  wires:
  In1/1 -> Terminator/1

== system lib_transmission2/hydraulic torque converter <htc> HEV/HTC for parallel HEV and Interface/model for parallel HEV/enhancedToWorkspace4 ==
  In1 : Inport
  Terminator : Terminator
  wires:
  In1/1 -> Terminator/1

== system lib_transmission2/hydraulic torque converter <htc> HEV/HTC for parallel HEV and Interface/model for parallel HEV/enhancedToWorkspace5 ==
  In1 : Inport
  Terminator : Terminator
  wires:
  In1/1 -> Terminator/1

== system lib_transmission2/hydraulic torque converter <htc> HEV/HTC for parallel HEV and Interface/model for parallel HEV/enhancedToWorkspace6 ==
  In1 : Inport
  Terminator : Terminator
  wires:
  In1/1 -> Terminator/1

== system lib_transmission2/hydraulic torque converter <htc> HEV/HTC for parallel HEV and Interface/model for parallel HEV/enhancedToWorkspace7 ==
  In1 : Inport
  Terminator : Terminator
  wires:
  In1/1 -> Terminator/1

== system lib_transmission2/hydraulic torque converter <htc> HEV/HTC for parallel HEV and Interface/model for parallel HEV/enhancedToWorkspace8 ==
  In1 : Inport
  Terminator : Terminator
  wires:
  In1/1 -> Terminator/1

== system lib_transmission2/hydraulic torque converter <htc> HEV/HTC for parallel HEV and Interface/model for parallel HEV/enhancedToWorkspace9 ==
  In1 : Inport
  Terminator : Terminator
  wires:
  In1/1 -> Terminator/1

== system lib_transmission2/hydraulic torque converter <htc> with pump loss/conventional HTC  and Interface/htc model/Block NOTES ==
  note: This block predicts the relative speed of the HTC input (pump) and output
      | (turbine).  Torque converter lockup is modeled.
      |
      | 1/24/00:tm updated gear_ratio flag to shifting flag
      |
      | 02/19/03: zz added pump loss
